simulink model "ccpi"  (R2023b)
settings: Solver=VariableStepAuto  StartTime=0.0  StopTime=10.0  RelTol=1e-3
values from neighbouring files (symbols this model uses):
  b = 50    [car.m]    (also in car_PID.m; car_PID_1.m; car_PI_1.m; car_PI_40.m)
  Ki = 50    [car_PID.m]    (also in car_PID_1.m = 1; car_PI_1.m = 1; car_PI_40.m = 40)
  Kp = 500    [car_PID.m]    (also in car_PID_1.m = 1; car_PI_1.m = 600; car_PI_40.m = 800; car_P_100.m = 100)
  m = 1000    [car.m]    (also in car_PID.m; car_PID_1.m; car_PI_1.m; car_PI_40.m)
  r = 10    [car.m]    (also in car_PID.m; car_PID_1.m; car_PI_1.m; car_PI_40.m)
settings Model: Creator=user  LastModifiedBy=user

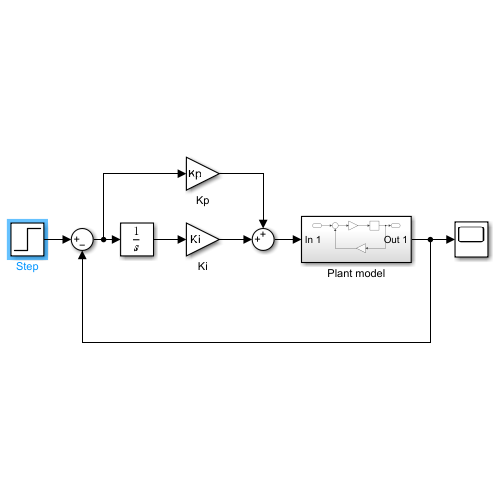
[thumbnail: Simulink's stored preview of the top-level diagram]
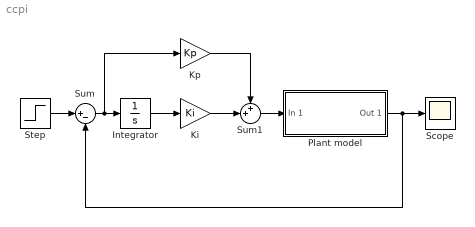
== system ccpi ==
  Integrator : Integrator
  Ki : Gain  Gain=Ki
  Kp : Gain  Gain=Kp
  Plant model : Subsystem
  Scope : Scope
  Step : Step  Time=0  After=r  SampleTime=0
  Sum : Sum  Inputs=|+-
  Sum1 : Sum  Inputs=++|
  wires:
  Plant model/1(Out 1) -> Scope/1, Sum/2
  Sum/1 -> Kp/1, Integrator/1
  Integrator/1 -> Ki/1
  Ki/1 -> Sum1/2
  Sum1/1 -> Plant model/1(In 1)
  Kp/1 -> Sum1/1
  Step/1 -> Sum/1

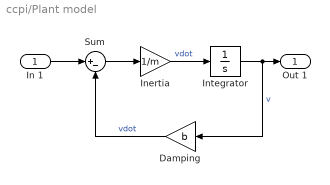
== system ccpi/Plant model ==
  In 1 : Inport
  Damping : Gain  Gain=b
  Inertia : Gain  Gain=1/m
  Integrator : Integrator
  Sum : Sum  Inputs=|+-
  Out 1 : Outport
  wires:
  Damping/1 -> Sum/2  "vdot"
  Sum/1 -> Inertia/1
  Inertia/1 -> Integrator/1  "vdot"
  In 1/1 -> Sum/1
  Integrator/1 -> Out 1/1, Damping/1  "v"
